simulink model "Pendulo_Doble"  (R2024a)
settings: Solver=VariableStepAuto  StartTime=0.0  StopTime=10.0  RelTol=1e-3
values from neighbouring files (symbols this model uses):
  g = 9.81    [PendDobParametros.m]
  l1 = 0.3    [PendDobParametros.m]
  l2 = 0.25    [PendDobParametros.m]
  m1 = 0.2    [PendDobParametros.m]
  m2 = 0.1    [PendDobParametros.m]
settings Model: Creator=Aguirre  LastModifiedBy=Aguirre

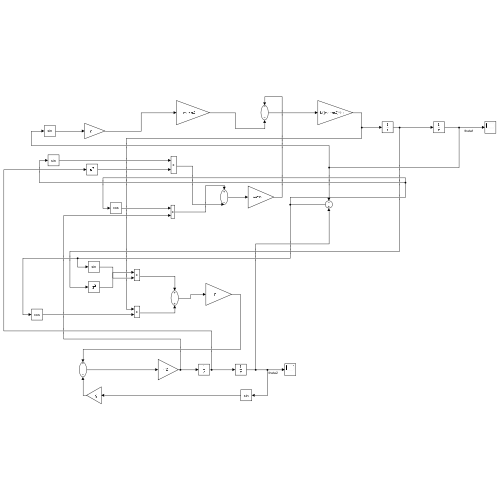
[thumbnail: Simulink's stored preview of the top-level diagram]
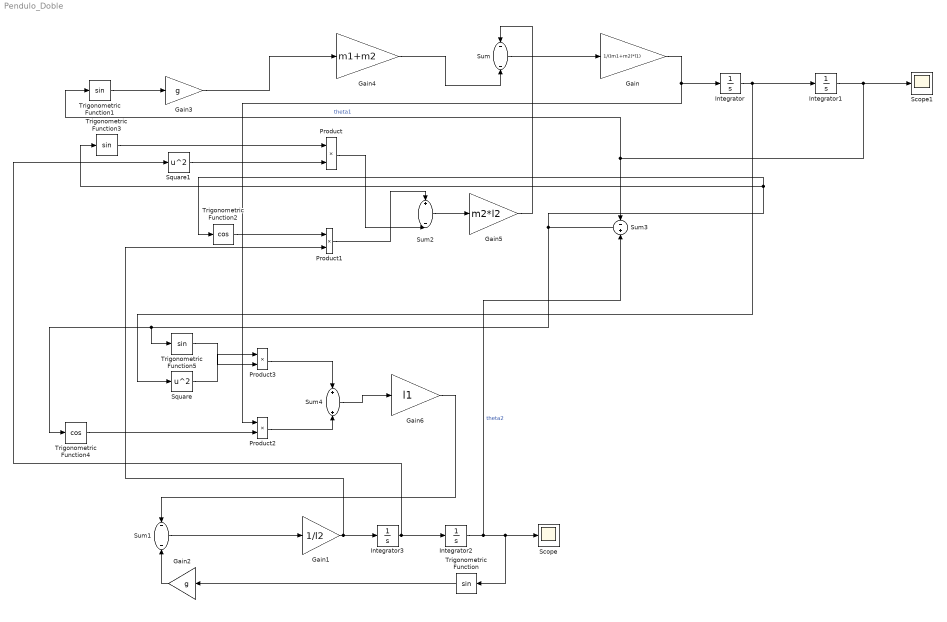
== system Pendulo_Doble ==
  Gain : Gain  Gain=1/((m1+m2)*l1)
  Gain1 : Gain  Gain=1/l2
  Gain2 : Gain  Gain=g
  Gain3 : Gain  Gain=g
  Gain4 : Gain  Gain=m1+m2
  Gain5 : Gain  Gain=m2*l2
  Gain6 : Gain  Gain=l1
  Integrator : Integrator
  Integrator1 : Integrator
  Integrator2 : Integrator  InitialCondition=(35*pi)/180
  Integrator3 : Integrator
  Product{,1..3} (4 alike) : Product
  Scope : Scope
  Scope1 : Scope
  Square : Math  Operator=square
  Square1 : Math  Operator=square
  Sum : Sum  Inputs=--
  Sum1 : Sum  Inputs=--
  Sum2 : Sum  Inputs=+-
  Sum3 : Sum  Inputs=-+
  Sum4 : Sum
  Trigonometric Function{,1,3,5} (4 alike) : Trigonometry
  Trigonometric Function2 : Trigonometry  Operator=cos
  Trigonometric Function4 : Trigonometry  Operator=cos
  wires:
  Sum2/1 -> Gain5/1
  Gain6/1 -> Sum1/1
  Square1/1 -> Product/2
  Square/1 -> Product3/1
  Trigonometric Function4/1 -> Product2/2
  Product3/1 -> Sum4/1
  Trigonometric Function1/1 -> Gain3/1
  Trigonometric Function5/1 -> Product3/2
  Trigonometric Function2/1 -> Product1/1
  Sum3/1 -> Trigonometric Function2/1, Trigonometric Function3/1, Trigonometric Function4/1, Trigonometric Function5/1
  Sum4/1 -> Gain6/1
  Integrator2/1 -> Scope/1, Trigonometric Function/1, Sum3/2  "theta2"
  Integrator1/1 -> Scope1/1, Trigonometric Function1/1, Sum3/1  "theta1"
  Gain5/1 -> Sum/1
  Gain3/1 -> Gain4/1
  Gain4/1 -> Sum/2
  Product1/1 -> Sum2/1
  Trigonometric Function/1 -> Gain2/1
  Sum/1 -> Gain/1
  Integrator/1 -> Integrator1/1, Square/1
  Integrator3/1 -> Integrator2/1, Square1/1
  Gain/1 -> Product2/1, Integrator/1
  Gain2/1 -> Sum1/2
  Product/1 -> Sum2/2
  Product2/1 -> Sum4/2
  Gain1/1 -> Integrator3/1, Product1/2
  Trigonometric Function3/1 -> Product/1
  Sum1/1 -> Gain1/1
